simulink library "ET3036TU_model_library_2020a_fix"  (R2020a)
settings: Solver=VariableStepAuto  StartTime=0.0  StopTime=10.0  RelTol=1e-3
values from neighbouring files (symbols this model uses):
  Data =     [Data.mat]
libraries: powerlib x21, simulink x13, powerlib_meascontrol x4
settings Model: Creator=Hazem  LastModifiedBy=simon
settings DebuggingCC: ArithmeticOperatorsInVariantConditions=warning
settings SFSimCC: CustomCodeUndefinedFunction=UseInterfaceOnly

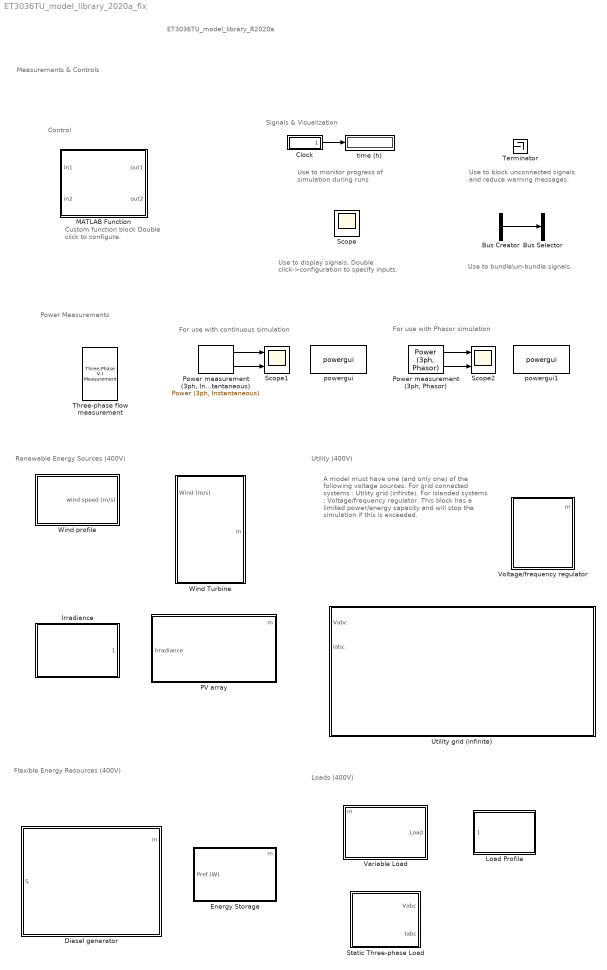
== system ET3036TU_model_library_2020a_fix ==
  note: Flexible Energy Resources (400V)
  note: Signals & Visualization
  note: Control
  note: Power Measurements
  note: ET3036TU_model_library_R2020a
  note: A model must have one (and only one) of the following voltage sources:
      |
      | For grid connected systems : Utility grid (infinite).
      |
      | For islanded systems : Voltage/frequency regulator. This block has a limited power/energy capacity and will stop the simulation if this is exceeded.
  note: Loads (400V)
  note: Utility (400V)
  note: Custom function block
      | Double click to configure.
  note: Use to display signals.
      | Double click->configuration to specify inputs.
  note: Use to bundle\un-bundle signals.
  note: Use to block unconnected signals
      | and reduce warning messages.
  note: Measurements & Controls
  note: Renewable Energy Sources (400V)
  note: For use with Phasor simulation
  note: For use with continuous simulation
  note: Use to monitor progress of
      | simulation during runs
  Bus Creator : BusCreator  Inputs=2
  Bus Selector : BusSelector  OutputSignals=Active power P (W),Reactive power Q (var)
  Clock : Subsystem
  Diesel generator : Subsystem  mask(Controllable Power Plant){Snom=15, Vnom=230*sqrt(3), fnom=50, Pfactor=1}
      mask prompts: Snom "Rated Power (MVA)"; Vnom "Rated phase-to-phase voltage (Vrms)"; fnom "Frequency (Hz)"; Pfactor "Power Factor (leading)"
      mask help: Implements a controllable (dispatchable) power plant with the required governer and excitation subsystems.
      mask Display:
      | image(imread('diesel.jpg'))
      | 
      | color('white')
      | port_label('RConn',1,'A')
      | port_label('RConn',2,'B')
      | port_label('RConn',3,'C')
      | port_label('output',1,'m')
      | 
      | color('black')
      | port_label('input',1,'  Sref (VA)')
  Energy Storage : Subsystem  mask(Grid-connected Energy Storage (PQ Model)){Vn=230*sqrt(3), Fn=50, PnomkW=100, kWh_Rated=500, Efficiency=96, LimitVec=[100 0], RechargeSOC=50, Precharge=100, autoRecharge=off, Initial_kWh_pc=50, PQvec=[0 0]}
      mask prompts: Vn "Nominal L-L Voltage [Vrms]"; Fn "Nominal Frequency [Hz]"; PnomkW "Rated Power [kW]"; kWh_Rated "Rated Capacity [kWh]"; Efficiency "Overall System Efficiency [%]"; LimitVec "Upper/Lower Charge Limits [%]"; RechargeSOC "SOC to Recharge [%]"; Precharge "Recharge Rate [% of Rated Power]"; autoRecharge "Enable Auto-Recharge"; Initial_kWh_pc "Initial State-of-Charge [0-100%]"; PQvec "Initial Active/Reactive Cmds"
      mask help:
      | The energy storage block models a generic grid-connected energy storage system (ESS), most commonly a battery system. This is a system-level model that does not contain any power electronics, but is useful for load flow, phasor, and hybrid phasor-EMT simulations. The inputs to this block are the commanded active and reactive power of the ESS.
      |
      | Note: Positive cmd indicates discharging (supply), negative cmd indicates charging (load).
      | Note: The initial active/reactive power commands must be specified for use for Load Flow analysis.
      mask init:
      | % Calculate Initial Conditions
      | Pnom = PnomkW*1e3;
      | P0 = -PQvec(1);  Q0 = -PQvec(2);
      | if abs(P0) > Pnom
      |     P0 = sign(P0)*Pnom;
      | end
      | 
      | % Calculate Q0 given Reactive Power Capability Curve
      | Qlim = sqrt(Pnom^2 - P0^2);
      | if Qlim > abs(Q0)
      |     Q0 = sign(Q0)*Qlim;
      | end
      | 
      | UpChrgLim = LimitVec(1);
      | LowChrgLim = LimitVec(2);
      | if Initial_kWh_pc > UpChrgLim && P0 < 0
      |     P0 = 0; Q0 = 0;
      | elseif Initial_kWh_pc < LowChrgLim && P0 > 0
      |     P0 = 0; Q0 = 0;
      | end
      mask DialogControl Container7 Prompt: Grid Connection Properties
      mask DialogControl Container11 Prompt: Charge/Discharge Controls
      mask DialogControl Container12 Prompt: Initial Conditions
      mask Display: image(imread('Battery.jpg'))
  Irradiance : Subsystem  mask(Irradiance profile){}
      mask help:
      | Automatically loads irradiance values from the local file 'Data.mat' (variable Data.solar).
      |
      | Expects hourly input irradiance values (W/m2).
      mask init:
      | load Data
      mask Display: plot(Data.solar.hour,Data.solar.direct+Data.solar.diffuse)
  Load Profile : Subsystem
      mask init:
      | load Data
      mask DialogControl DescGroupVar Prompt: Load Profile
      mask DialogControl DescTextVar Prompt: Automatically loads Consumption values from the local file 'Data.mat' (variable Data.varload).
      mask DialogControl Control2 Prompt: Expects per-minute active power consumption values (W).
      mask Display: plot(Data.varload.minute,Data.varload.load)
  MATLAB Function : MATLAB Function  TreatAsAtomicUnit=on
  "PV array " : Subsystem  mask(PV farm){Efficiency=0.2, Area=100, Vnom=230*sqrt(3), fnom=50}
      mask prompts: Efficiency "Total efficiency (fraction)"; Area "Area (m2)"; Vnom "Rated phase-to-phase voltage (Vrms)"; fnom "Rated frequency (Hz):"
      mask help: The product of the efficiency, the area covered by the PV farm and the irradiance in W/m2 will give you the power generated by the PV farm.
      mask Display:
      | color('white')
      | image(imread('pv.jpg'))
      | 
      | color('black')
      | port_label('RConn',1,'A')
      | port_label('RConn',2,'B')
      | port_label('RConn',3,'C')
      | port_label('output',1,'m')
      | 
      | port_label('input',1,'Irradiance (W/m2)')
  "Power measurement (3ph, Instantaneous)" : powerlib_meascontrol/Measurements/Power (3ph, Instantaneous)
  "Power measurement (3ph, Phasor)" : powerlib_meascontrol/Measurements/Power (3ph, Phasor)
      settings: SourceProductBaseCode=PS
  Scope : Scope  NumInputPorts=2
  Scope1 : Scope  NumInputPorts=2
  Scope2 : Scope  NumInputPorts=2
  Static Three-phase Load : Subsystem  mask(Static Three-phase Load){Vnom=230*sqrt(3), fnom=50, Prated=100}
      mask prompts: Vnom "Nominal phase-to-phase voltage Vn (Vrms)"; fnom "Nominal frequency fn (Hz):"; Prated "Active power P (kW):"
      mask help:
      | Implements a three-phase resistive load.
      |
      | Adjust nominal voltage and frequency according to system configuration.
      |
      | Specify rated power consumption.
      mask Display: image(imread('Res.jpg'))
  Terminator : Terminator
  Three-phase flow measurement : powerlib/Measurements/Three-Phase V-I Measurement  VoltageMeasurement=phase-to-ground  SetLabelV=off  LabelV=Vabc  Vpu=off  VpuLL=off  CurrentMeasurement=yes  SetLabelI=off  LabelI=Iabc  Ipu=off  Pbase=100e6  Vbase=500e3  OutputType=Complex  PhasorSimulation=on  PSBequivalent=0
  Utility grid (infinite) : Subsystem  mask(Utility Distribution Substation){Vgrid=230*sqrt(3), fnom=50}
      mask prompts: Vgrid "Grid phase-to-phase  voltage (Vrms)"; fnom "Nominal frequency (Hz):"
      mask help:
      | Implements a grid connection with finite capacity.
      |
      | Supports two-way power flow, set voltages and frequency according to system configuration.
      |
      | Adjust Nominal Power.
      mask Display:
      | image(imread('powersystem.jpg'))
      | 
      | color('white')
      | port_label('RConn',1,'A')
      | port_label('RConn',2,'B')
      | port_label('RConn',3,'C')
      | port_label('output',1,'Vabc')
      | port_label('output',2,'Iabc')
  Variable Load : Subsystem  mask(Variable Load (PQ Model)){Vn=230*sqrt(3), Fn=50, PF=1, Load0=0}
      mask prompts: Vn "Nominal L-L Voltage [Vrms]"; Fn "Nominal Frequency [Hz]"; PF "Power Factor [0 to 1]"; Load0 "Initial Load [W]"
      mask help:
      | The Variable Load block is a lumped approximation for a distribution feeder. For non-unity power factor loads, the input (active power) is scaled accordingly to generate a desired load.
      |
      | Note: The initial input load must be specified for use for Load Flow analysis.
      mask init:
      | P0 = Load0;
      | Q0 = Load0*sqrt(1/PF-1);
      mask Display:
      | image(imread('Residential.jpg'))
      | color('white')
      | port_label('input',1,'Load (W)')
      | port_label('output',1,'m')
      | port_label('Rconn',1,'A')
      | port_label('Rconn',2,'B')
      | port_label('Rconn',3,'C')
  Voltage/frequency regulator : Subsystem  mask{E_max=1e3, Vnom=230*sqrt(3), fnom=50}
      mask prompts: E_max "Rated energy reserve (Wh)"; Vnom "Nominal L-L Voltage (Vrms)"; fnom "Nominal Frequency (Hz)"
      mask Display: image(imread('powerlib_icon.jpg'))
  "Wind Turbine " : Subsystem  mask{Unom=15, Umax=25, Umin=5, Pselect=1: Simple Cubic Power, fnom=50, Vnom=230*sqrt(3), Pnom=20, rp=5, Cp=16/27, rho=1.225, Uvec=[1:1:30], Pvec=[0,0,0,0,21359.3750000000,58193.5000000000,104316.125000000,157104.500000000,213935.875000000,272187.500000000,329236.625000000,382460.500000000,429236.375000000,466941.500000000,492953.125000000,500000,500000,500000,500000,500000,500000,500000,500000,500000,500000,0,0,0,0,0], Tp=0.1, Tq=1, ReactP=0}
      mask prompts: Unom "Nominal Wind Speed [m/s]"; Umax "Maximum Operating Wind [m/s]"; Umin "Minimum Operating Wind [m/s]"; Pselect "Wind Turbine Power Model"; fnom "Nominal frequency (Hz):"; Vnom "Nominal phae-to-phase voltage (Vrms)"; Pnom "Nominal Power, [kW]"; rp "Blade Radius, r [m]"; Cp "Performance Coefficient, Cp"; rho "Air Density, rho [kg/m^3]"; Uvec "Wind Vec [m/s]"; Pvec "Power Vec [W]"; Tp "Active Power Dynamics, Tp [s]"; Tq "Reactive Power Dynamics, Tq [s]"; ReactP "Reactive Power Percentage [%]"
      mask help:
      | Simple Wind Turbine that serves as an Active and Reactive Power Source depending on the Wind Power Curve.
      |
      | The Wind Turbine Power Curve can be defined by one of three models:
      | 1: Simple cubic power curve
      | 2: Physical wind turbine parameters
      | 3: Look-up table (from a wind turbine data sheet).
      |
      | The 'General' and 'Dynamics' tabs apply to all models.
      mask init:
      | A = pi*rp^2;
      | 
      | if Pselect == 1,
      |     Pmax = Pnom*1e3;
      | elseif Pselect == 2,
      |     Pmax = 1/2*rho*Cp*A*Umax^3;
      | else
      |     Pmax = max(Pvec);
      | end
      | Qmax = (ReactP/100)*Pmax;
      mask TypeOptions Pselect: 1: Simple Cubic Power | 2: Physical parameters | 3: Look-up Fit
      mask DialogControl Container4 Prompt: General
      mask DialogControl Container16 Prompt: Turbine
      mask DialogControl Container10 Prompt: Electrical
      mask DialogControl Container12 Prompt: 1: Cubic
      mask DialogControl Container9 Prompt: 2: Physical
      mask DialogControl Container7 Prompt: 3: Lookup
      mask DialogControl Container8 Prompt: Dynamics
      mask Display:
      | image(imread('eolienne.bmp'))
      | 
      | color('white')
      | port_label('LConn',1,'A')
      | port_label('LConn',2,'B')
      | port_label('LConn',3,'C')
      | 
      | color('blue')
      | port_label('output',1,'m')
      | port_label('input',1,'Wind (m/s)')
  Wind profile : Subsystem  mask(Wind profile){}
      mask help:
      | Automatically loads wind speeds from the local file 'Data.mat' (variable Data.wind).
      |
      | Expects hourly input wind speeds (m/s).
      mask init:
      | load Data
      mask Display: plot(Data.wind.hour,Data.wind.speed)
  powergui : powerlib/powergui  Priority=1  SimulationMode=Discrete  SampleTime=1e-3  frequency=60  Iterations=50  frequencyindice=60  Pbase=100e6  ErrMax=1e-4  UnitsV=kV  UnitsW=MW  buscounter=0  FunctionMessages=off  echomessages=off  EnableUseOfTLC=off  CurrentSourceSwitches=off  DisableSnubberDevices=off  DisableRonSwitches=off  DisableVfSwitches=off  DisplayEquations=off  AutomaticDiscreteSolvers=off  SolverType=Tustin/Backward Euler (TBE)  Interpol=off  ExternalGateDelay=off  methode=off  Ts=100  x0status=blocks  SPID=on  SwTol=0  HookPort=off  NonlinearTolerance=0  nMaxIteration=15  ContinueOnMaxIteration=off  RestoreLinks=warning  ResistiveCurrentMeasurement=off  Frange=[0:2:500]  Ylog=off  Xlog=on  ShowGrid=off  save=off  variable=ZData  structure=0  ZoomFFT=off  StartTime=0.0  cycles=1  DisplayStyle=1  fundamental=60  FreqAxis=off  MaxFrequency=1000  frequencyindicesteady=1  RmsSteady=1  display=off
  powergui1 : powerlib/powergui  Priority=1  SimulationMode=Phasor  SampleTime=50e-6  frequency=50  Iterations=50  frequencyindice=60  Pbase=100e6  ErrMax=1e-4  UnitsV=kV  UnitsW=MW  buscounter=0  FunctionMessages=off  echomessages=off  EnableUseOfTLC=off  CurrentSourceSwitches=off  DisableSnubberDevices=off  DisableRonSwitches=off  DisableVfSwitches=off  DisplayEquations=off  AutomaticDiscreteSolvers=off  SolverType=Tustin/Backward Euler (TBE)  Interpol=off  ExternalGateDelay=off  methode=off  Ts=100  x0status=blocks  SPID=on  SwTol=0  HookPort=off  NonlinearTolerance=0  nMaxIteration=15  ContinueOnMaxIteration=off  RestoreLinks=warning  ResistiveCurrentMeasurement=off  Frange=[0:2:500]  Ylog=off  Xlog=on  ShowGrid=off  save=off  variable=ZData  structure=0  ZoomFFT=off  StartTime=0.0  cycles=1  DisplayStyle=1  fundamental=60  FreqAxis=off  MaxFrequency=1000  frequencyindicesteady=1  RmsSteady=1  display=off
  time (h) : Display
      settings: Format=bank
  wires:
  "Power measurement (3ph, Phasor)"/1 -> Scope2/1
  "Power measurement (3ph, Phasor)"/2 -> Scope2/2
  "Power measurement (3ph, Instantaneous)"/1 -> Scope1/1
  "Power measurement (3ph, Instantaneous)"/2 -> Scope1/2
  Clock/1(" ") -> time (h)/1
  Bus Creator/1 -> Bus Selector/1

== system ET3036TU_model_library_2020a_fix/Clock ==
  Clock : Clock
  Gain : Gain  Gain=1/(60*60)
  " " : Outport  VectorParamsAs1DForOutWhenUnconnected=off
  wires:
  Gain/1 -> " "/1
  Clock/1 -> Gain/1

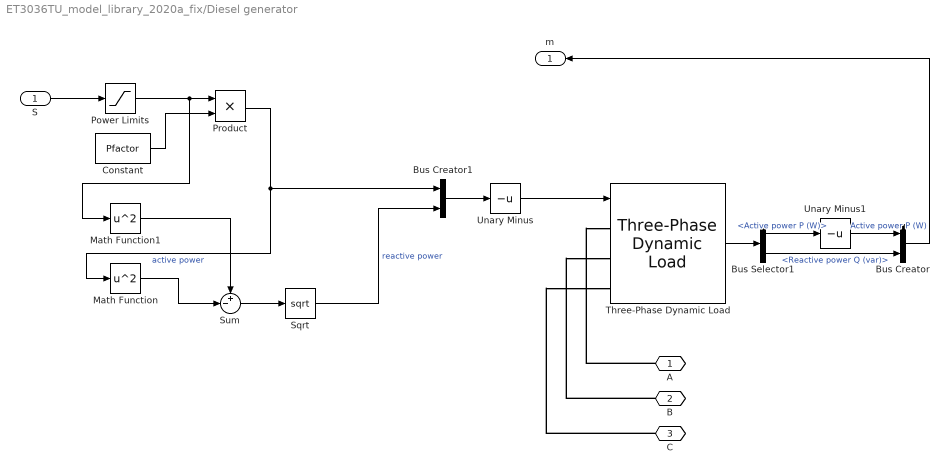
== system ET3036TU_model_library_2020a_fix/Diesel generator ==
  S : Inport
  Bus Creator : BusCreator  Inputs=2
  Bus Creator1 : BusCreator  Inputs=2
  Bus Selector1 : BusSelector  OutputSignals=Active power P (W),Reactive power Q (var)
  Constant : Constant  Value=Pfactor
  Math Function : Math  Operator=square  SignedPower=on  SaturateOnIntegerOverflow=on
  Math Function1 : Math  Operator=square  SignedPower=on  SaturateOnIntegerOverflow=on
  Power Limits : Saturate  UpperLimit=Snom*1e6  LowerLimit=0
  Product : Product
  Sqrt : Sqrt  SaturateOnIntegerOverflow=on
  Sum : Sum  Inputs=+-|
  Three-Phase Dynamic Load : powerlib/Elements/Three-Phase Dynamic Load  NominalVoltage=[Vnom fnom]  ActiveReactivePowers=[0 0]  PositiveSequence=[Vnom 0]  ExternalControl=on  NpNq=[1.3 2]  TimeConstants="[0  0  0  0]"  MinimumVoltage=0.7  Tfilter=1e-4  LoadFlowParameters=[4,0,0,0,0]
      settings: SourceProductBaseCode=PS
  Unary Minus : UnaryMinus
  Unary Minus1 : UnaryMinus
  A : PMIOPort  Side=Right
  B : PMIOPort  Port=2  Side=Right
  C : PMIOPort  Port=3  Side=Right
  m : Outport  VectorParamsAs1DForOutWhenUnconnected=off
  wires:
  Constant/1 -> Product/2
  Math Function1/1 -> Sum/1
  Math Function/1 -> Sum/2
  Product/1 -> Math Function/1, Bus Creator1/1  "active power"
  S/1 -> Power Limits/1
  Sum/1 -> Sqrt/1
  Power Limits/1 -> Math Function1/1, Product/1
  Sqrt/1 -> Bus Creator1/2  "reactive power"
  Bus Selector1/2 -> Bus Creator/2  "<Reactive power Q (var)>"
  Three-Phase Dynamic Load/1 -> Bus Selector1/1
  Bus Selector1/1 -> Unary Minus1/1  "<Active power P (W)>"
  Unary Minus1/1 -> Bus Creator/1  "Active power P (W)"
  Bus Creator/1 -> m/1
  Bus Creator1/1 -> Unary Minus/1
  Unary Minus/1 -> Three-Phase Dynamic Load/1
  connections:
  A/RConn1 -- Three-Phase Dynamic Load/LConn1
  B/RConn1 -- Three-Phase Dynamic Load/LConn2
  C/RConn1 -- Three-Phase Dynamic Load/LConn3

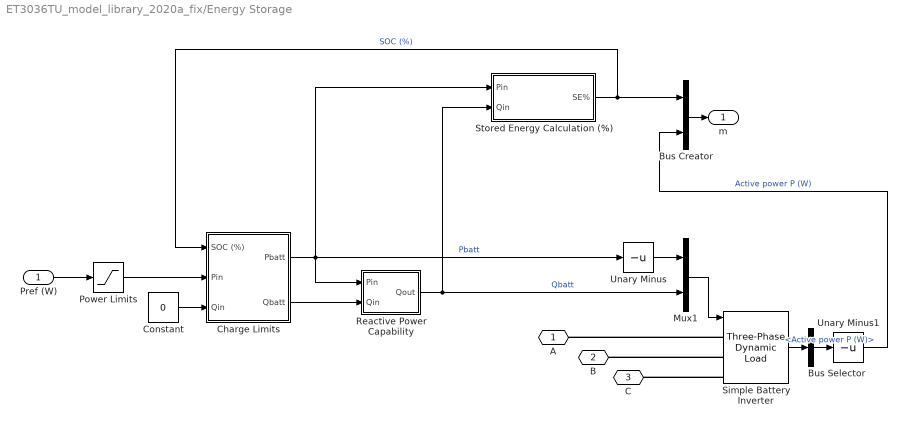
== system ET3036TU_model_library_2020a_fix/Energy Storage ==
  Pref (W) : Inport
  Bus Creator : BusCreator  Inputs=2
  Bus Selector : BusSelector  OutputSignals=Active power P (W)
  Charge Limits : Subsystem
  Constant : Constant  Value=0
  Mux1 : Mux  Inputs=2
  Power Limits : Saturate  UpperLimit=Pnom  LowerLimit=-Pnom
  Reactive Power Capability : Subsystem
  Simple Battery Inverter : powerlib/Elements/Three-Phase Dynamic Load  NominalVoltage=[Vn Fn]  ActiveReactivePowers=[0 0]  PositiveSequence=[Vn 0]  ExternalControl=on  NpNq=[1.3 2]  TimeConstants="[0  0  0  0]"  MinimumVoltage=0.7  Tfilter=1e-4  LoadFlowParameters=[4,0,0,0,0]
      settings: SourceProductBaseCode=PS
  Stored Energy Calculation (%) : Subsystem
  Unary Minus : UnaryMinus
  Unary Minus1 : UnaryMinus
  A : PMIOPort  Side=Right
  B : PMIOPort  Port=2  Side=Right
  C : PMIOPort  Port=3  Side=Right
  m : Outport  VectorParamsAs1DForOutWhenUnconnected=off
  wires:
  Unary Minus/1 -> Mux1/1
  Mux1/1 -> Simple Battery Inverter/1
  Simple Battery Inverter/1 -> Bus Selector/1
  Reactive Power Capability/1(Qout) -> Stored Energy Calculation (%)/2(Qin), Mux1/2  "Qbatt"
  Pref (W)/1 -> Power Limits/1
  Bus Creator/1 -> m/1
  Stored Energy Calculation (%)/1(SE%) -> Charge Limits/1(SOC (%)), Bus Creator/1  "SOC (%)"
  Charge Limits/1(Pbatt) -> Stored Energy Calculation (%)/1(Pin), Unary Minus/1, Reactive Power Capability/1(Pin)  "Pbatt"
  Power Limits/1 -> Charge Limits/2(Pin)
  Constant/1 -> Charge Limits/3(Qin)
  Charge Limits/2(Qbatt) -> Reactive Power Capability/2(Qin)
  Bus Selector/1 -> Unary Minus1/1  "<Active power P (W)>"
  Unary Minus1/1 -> Bus Creator/2  "Active power P (W)"
  connections:
  Simple Battery Inverter/LConn2 -- B/RConn1
  Simple Battery Inverter/LConn3 -- C/RConn1
  Simple Battery Inverter/LConn1 -- A/RConn1

== system ET3036TU_model_library_2020a_fix/Irradiance ==
  Add : Sum
  Add1 : Sum
  Clock1 : Clock
  Constant1 : Constant
  Diffuse irradiance series : Lookup_n-D  NumberOfTableDimensions=1  BreakpointsForDimension1=Data.solar.hour  BeginIndexSearchUsingPreviousIndexResult=on  Table=Data.solar.diffuse  InternalRulePriority=Speed  RndMeth=Simplest  InputSameDT=on
  Direct irradiance series : Lookup_n-D  NumberOfTableDimensions=1  BreakpointsForDimension1=Data.solar.hour  BeginIndexSearchUsingPreviousIndexResult=on  Table=Data.solar.direct  InternalRulePriority=Speed  RndMeth=Simplest  InputSameDT=on
  Second-->Hour : Gain  Gain=1/(60*60)
  " " : Outport  VectorParamsAs1DForOutWhenUnconnected=off
  wires:
  Constant1/1 -> Add/2
  Add/1 -> Direct irradiance series/1, Diffuse irradiance series/1  "Simulation hour"
  Clock1/1 -> Second-->Hour/1
  Second-->Hour/1 -> Add/1
  Diffuse irradiance series/1 -> Add1/1
  Direct irradiance series/1 -> Add1/2
  Add1/1 -> " "/1  "Simulation hour"

== system ET3036TU_model_library_2020a_fix/Load Profile ==
  Add : Sum
  Clock1 : Clock
  Constant1 : Constant
  Second-->Minute : Gain  Gain=1/(60)
  load profile series : Lookup_n-D  NumberOfTableDimensions=1  BreakpointsForDimension1=Data.varload.minute  BeginIndexSearchUsingPreviousIndexResult=on  Table=Data.varload.load  InternalRulePriority=Speed  RndMeth=Simplest  InputSameDT=on
  " " : Outport  VectorParamsAs1DForOutWhenUnconnected=off
  wires:
  Constant1/1 -> Add/2
  Add/1 -> load profile series/1  "Minute"
  load profile series/1 -> " "/1
  Clock1/1 -> Second-->Minute/1
  Second-->Minute/1 -> Add/1

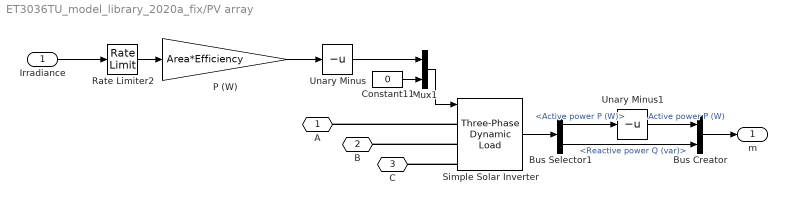
== system ET3036TU_model_library_2020a_fix/PV array  ==
  Irradiance : Inport
  Bus Creator : BusCreator  Inputs=2
  Bus Selector1 : BusSelector  OutputSignals=Active power P (W),Reactive power Q (var)
  Constant11 : Constant  Value=0
  Mux1 : Mux  Inputs=2
  P (W) : Gain  Gain=Area*Efficiency
  Rate Limiter2 : RateLimiter  RisingSlewLimit=1e4  FallingSlewLimit=-1e4  SampleTimeMode=inherited
  Simple Solar Inverter : powerlib/Elements/Three-Phase Dynamic Load  NominalVoltage=[Vnom fnom]  ActiveReactivePowers=[0 0]  PositiveSequence=[Vnom 0]  ExternalControl=on  NpNq=[1.3 2]  TimeConstants="[0  0  0  0]"  MinimumVoltage=0.7  Tfilter=1e-4  LoadFlowParameters=[4,0,0,0,0]
      settings: SourceProductBaseCode=PS
  Unary Minus : UnaryMinus
  Unary Minus1 : UnaryMinus
  A : PMIOPort  Side=Right
  B : PMIOPort  Port=2  Side=Right
  C : PMIOPort  Port=3  Side=Right
  m : Outport  VectorParamsAs1DForOutWhenUnconnected=off
  wires:
  Rate Limiter2/1 -> P (W)/1
  Constant11/1 -> Mux1/2
  Mux1/1 -> Simple Solar Inverter/1
  Unary Minus/1 -> Mux1/1
  Simple Solar Inverter/1 -> Bus Selector1/1
  Bus Selector1/1 -> Unary Minus1/1  "<Active power P (W)>"
  P (W)/1 -> Unary Minus/1
  Irradiance/1 -> Rate Limiter2/1
  Unary Minus1/1 -> Bus Creator/1  "Active power P (W)"
  Bus Selector1/2 -> Bus Creator/2  "<Reactive power Q (var)>"
  Bus Creator/1 -> m/1
  connections:
  Simple Solar Inverter/LConn2 -- B/RConn1
  Simple Solar Inverter/LConn1 -- A/RConn1
  Simple Solar Inverter/LConn3 -- C/RConn1

== system ET3036TU_model_library_2020a_fix/Static Three-phase Load ==
  Static Load : powerlib/Elements/Three-Phase Series RLC Load  LConnTagsString=A|B|C  Configuration=Y (grounded)  NominalVoltage=Vnom  Vabc=[1e3 1e3 1e3]  Vabcp=[1e3 1e3 1e3]  NominalFrequency=fnom  UnbalancedPower=off  ActivePower=Prated*1e3  InductivePower=0  CapacitivePower=0  Pabc=[10e3 9e3 11e3]  QLabc=[100 90 110]  QCabc=[100 90 110]  Pabcp=[10e3 9e3 11e3]  QLabcp=[100 90 110]  QCabcp=[100 90 110]  Measurements=None  LoadType=constant Z
  V-I Measurement : powerlib/Measurements/Three-Phase V-I Measurement  VoltageMeasurement=phase-to-ground  SetLabelV=off  LabelV=Vabc  Vpu=off  VpuLL=off  CurrentMeasurement=yes  SetLabelI=off  LabelI=Iabc  Ipu=off  Pbase=100e6  Vbase=500e3  OutputType=Complex  PhasorSimulation=on  PSBequivalent=0
  A : PMIOPort  Side=Left
  B : PMIOPort  Port=2  Side=Left
  C : PMIOPort  Port=3  Side=Left
  Vabc : Outport  VectorParamsAs1DForOutWhenUnconnected=off
  Iabc : Outport  Port=2  VectorParamsAs1DForOutWhenUnconnected=off
  wires:
  V-I Measurement/1 -> Vabc/1
  V-I Measurement/2 -> Iabc/1
  connections:
  Static Load/LConn1 -- V-I Measurement/LConn1
  V-I Measurement/RConn1 -- A/RConn1
  V-I Measurement/LConn2 -- Static Load/LConn2
  V-I Measurement/RConn3 -- C/RConn1
  Static Load/LConn3 -- V-I Measurement/LConn3
  V-I Measurement/RConn2 -- B/RConn1

== system ET3036TU_model_library_2020a_fix/Utility grid (infinite) ==
  AC Voltage Source : powerlib/Electrical Sources/AC Voltage Source  Amplitude=Vgrid*sqrt(2)/sqrt(3)  Phase=0  Frequency=fnom  SampleTime=0  Measurements=None  BusType=swing  Pref=10e3  Qref=0  Qmin=-inf  Qmax=+inf
  AC Voltage Source1 : powerlib/Electrical Sources/AC Voltage Source  Amplitude=Vgrid*sqrt(2)/sqrt(3)  Phase=-120  Frequency=fnom  SampleTime=0  Measurements=None  BusType=swing  Pref=10e3  Qref=0  Qmin=-inf  Qmax=+inf
  AC Voltage Source2 : powerlib/Electrical Sources/AC Voltage Source  Amplitude=Vgrid*sqrt(2)/sqrt(3)  Phase=120  Frequency=fnom  SampleTime=0  Measurements=None  BusType=swing  Pref=10e3  Qref=0  Qmin=-inf  Qmax=+inf
  Ground : powerlib/Elements/Ground  LConnTagsString=a
  V-I Measurement : powerlib/Measurements/Three-Phase V-I Measurement  VoltageMeasurement=phase-to-ground  SetLabelV=off  LabelV=Vabc  Vpu=off  VpuLL=off  CurrentMeasurement=yes  SetLabelI=off  LabelI=Iabc  Ipu=off  Pbase=100e6  Vbase=500e3  OutputType=Complex  PhasorSimulation=off  PSBequivalent=0
  A : PMIOPort  Side=Right
  B : PMIOPort  Port=2  Side=Right
  C : PMIOPort  Port=3  Side=Right
  Vabc : Outport  VectorParamsAs1DForOutWhenUnconnected=off
  Iabc : Outport  Port=2  VectorParamsAs1DForOutWhenUnconnected=off
  wires:
  V-I Measurement/2 -> Iabc/1  "Iabc"
  V-I Measurement/1 -> Vabc/1  "Vabc"
  connections:
  Ground/LConn1 -- AC Voltage Source2/LConn1 -- AC Voltage Source1/LConn1 -- AC Voltage Source/LConn1
  AC Voltage Source1/RConn1 -- V-I Measurement/LConn2
  AC Voltage Source/RConn1 -- V-I Measurement/LConn1
  AC Voltage Source2/RConn1 -- V-I Measurement/LConn3
  B/RConn1 -- V-I Measurement/RConn2
  C/RConn1 -- V-I Measurement/RConn3
  V-I Measurement/RConn1 -- A/RConn1

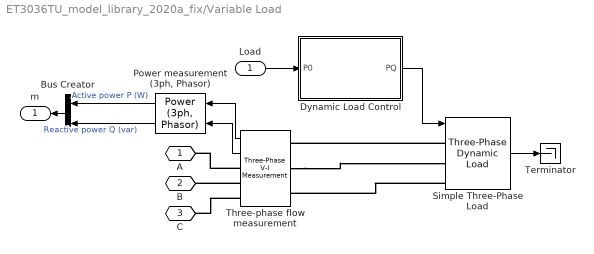
== system ET3036TU_model_library_2020a_fix/Variable Load ==
  Load : Inport
  Bus Creator : BusCreator  Inputs=2
  Dynamic Load Control : Subsystem
  "Power measurement (3ph, Phasor)" : powerlib_meascontrol/Measurements/Power (3ph, Phasor)
      settings: SourceProductBaseCode=PS
  Simple Three-Phase Load : powerlib/Elements/Three-Phase Dynamic Load  NominalVoltage=[Vn Fn]  ActiveReactivePowers=[0 0]  PositiveSequence=[Vn 0]  ExternalControl=on  NpNq=[1.3 2]  TimeConstants="[0  0  0  0]"  MinimumVoltage=0.7  Tfilter=1e-4  LoadFlowParameters=[4,0,0,0,0]
      settings: SourceProductBaseCode=PS
  Terminator : Terminator
  Three-phase flow measurement : powerlib/Measurements/Three-Phase V-I Measurement  VoltageMeasurement=phase-to-ground  SetLabelV=off  LabelV=Vabc  Vpu=off  VpuLL=off  CurrentMeasurement=yes  SetLabelI=off  LabelI=Iabc  Ipu=off  Pbase=100e6  Vbase=500e3  OutputType=Complex  PhasorSimulation=on  PSBequivalent=0
  A : PMIOPort  Side=Right
  B : PMIOPort  Port=2  Side=Right
  C : PMIOPort  Port=3  Side=Right
  m : Outport  VectorParamsAs1DForOutWhenUnconnected=off
  wires:
  "Power measurement (3ph, Phasor)"/2 -> Bus Creator/2  "Reactive power Q (var)"
  "Power measurement (3ph, Phasor)"/1 -> Bus Creator/1  "Active power P (W)"
  Bus Creator/1 -> m/1
  Three-phase flow measurement/1 -> "Power measurement (3ph, Phasor)"/1
  Three-phase flow measurement/2 -> "Power measurement (3ph, Phasor)"/2
  Load/1 -> Dynamic Load Control/1(P0)
  Dynamic Load Control/1(PQ) -> Simple Three-Phase Load/1
  Simple Three-Phase Load/1 -> Terminator/1
  connections:
  Three-phase flow measurement/RConn3 -- C/RConn1
  Three-phase flow measurement/RConn2 -- B/RConn1
  Three-phase flow measurement/RConn1 -- A/RConn1
  Simple Three-Phase Load/LConn3 -- Three-phase flow measurement/LConn3
  Simple Three-Phase Load/LConn1 -- Three-phase flow measurement/LConn1
  Three-phase flow measurement/LConn2 -- Simple Three-Phase Load/LConn2

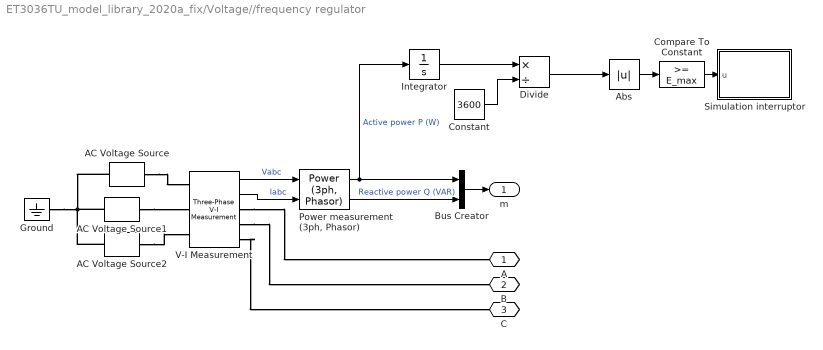
== system ET3036TU_model_library_2020a_fix/Voltage//frequency regulator ==
  AC Voltage Source : powerlib/Electrical Sources/AC Voltage Source  Amplitude=Vnom*sqrt(2)/sqrt(3)  Phase=0  Frequency=fnom  SampleTime=0  Measurements=None  BusType=swing  Pref=10e3  Qref=0  Qmin=-inf  Qmax=+inf
  AC Voltage Source1 : powerlib/Electrical Sources/AC Voltage Source  Amplitude=Vnom*sqrt(2)/sqrt(3)  Phase=-120  Frequency=fnom  SampleTime=0  Measurements=None  BusType=swing  Pref=10e3  Qref=0  Qmin=-inf  Qmax=+inf
  AC Voltage Source2 : powerlib/Electrical Sources/AC Voltage Source  Amplitude=Vnom*sqrt(2)/sqrt(3)  Phase=120  Frequency=fnom  SampleTime=0  Measurements=None  BusType=swing  Pref=10e3  Qref=0  Qmin=-inf  Qmax=+inf
  Abs : Abs
  Bus Creator : BusCreator  Inputs=2
  Compare To Constant : simulink/Logic and Bit Operations/Compare To Constant  relop=>=  const=E_max  OutDataTypeStr=boolean
  Constant : Constant  Value=3600
  Divide : Product  Inputs=*/
  Ground : powerlib/Elements/Ground  LConnTagsString=a
  Integrator : Integrator
  "Power measurement (3ph, Phasor)" : powerlib_meascontrol/Measurements/Power (3ph, Phasor)
      settings: SourceProductBaseCode=PS
  Simulation interruptor : MATLAB Function  TreatAsAtomicUnit=on
  V-I Measurement : powerlib/Measurements/Three-Phase V-I Measurement  VoltageMeasurement=phase-to-ground  SetLabelV=off  LabelV=Vabc  Vpu=off  VpuLL=off  CurrentMeasurement=yes  SetLabelI=off  LabelI=Iabc  Ipu=off  Pbase=100e6  Vbase=500e3  OutputType=Complex  PhasorSimulation=on  PSBequivalent=0
  A : PMIOPort  Side=Right
  B : PMIOPort  Port=2  Side=Right
  C : PMIOPort  Port=3  Side=Right
  m : Outport
  wires:
  "Power measurement (3ph, Phasor)"/1 -> Integrator/1, Bus Creator/1  "Active power P (W)"
  Integrator/1 -> Divide/1
  Abs/1 -> Compare To Constant/1
  V-I Measurement/1 -> "Power measurement (3ph, Phasor)"/1  "Vabc"
  V-I Measurement/2 -> "Power measurement (3ph, Phasor)"/2  "Iabc"
  "Power measurement (3ph, Phasor)"/2 -> Bus Creator/2  "Reactive power Q (VAR)"
  Bus Creator/1 -> m/1
  Compare To Constant/1 -> Simulation interruptor/1(u)
  Constant/1 -> Divide/2
  Divide/1 -> Abs/1
  connections:
  V-I Measurement/RConn3 -- C/RConn1
  AC Voltage Source/RConn1 -- V-I Measurement/LConn1
  AC Voltage Source1/RConn1 -- V-I Measurement/LConn2
  V-I Measurement/RConn1 -- A/RConn1
  AC Voltage Source2/RConn1 -- V-I Measurement/LConn3
  Ground/LConn1 -- AC Voltage Source/LConn1 -- AC Voltage Source1/LConn1 -- AC Voltage Source2/LConn1
  V-I Measurement/RConn2 -- B/RConn1

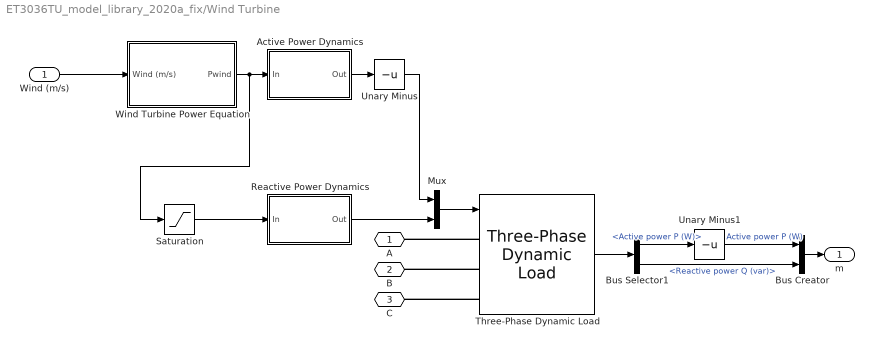
== system ET3036TU_model_library_2020a_fix/Wind Turbine  ==
  Wind (m/s) : Inport
  Active Power Dynamics : Subsystem  VariantControl=T6NotZero
      mask Display: disp('1 / (1 + s T_P)','texmode','on');
  Bus Creator : BusCreator  Inputs=2
  Bus Selector1 : BusSelector  OutputSignals=Active power P (W),Reactive power Q (var)
  Mux : Mux  Inputs=2
  Reactive Power Dynamics : Subsystem  VariantControl=T6NotZero
      mask Display: disp('1 / (1 + s T_Q)','texmode','on');
  Saturation : Saturate  UpperLimit=Qmax  LowerLimit=-Qmax
  Three-Phase Dynamic Load : powerlib/Elements/Three-Phase Dynamic Load  NominalVoltage=[Vnom fnom]  ActiveReactivePowers=[0 0]  PositiveSequence=[Vnom 0]  ExternalControl=on  NpNq=[1.3 2]  TimeConstants="[0  0  0  0]"  MinimumVoltage=0.7  Tfilter=1e-4  LoadFlowParameters=[4,0,0,0,0]
      settings: SourceProductBaseCode=PS
  Unary Minus : UnaryMinus
  Unary Minus1 : UnaryMinus
  Wind Turbine Power Equation : Subsystem
  A : PMIOPort  Side=Left
  B : PMIOPort  Port=2  Side=Left
  C : PMIOPort  Port=3  Side=Left
  m : Outport  VectorParamsAs1DForOutWhenUnconnected=off
  wires:
  Bus Selector1/2 -> Bus Creator/2  "<Reactive power Q (var)>"
  Bus Creator/1 -> m/1
  Unary Minus1/1 -> Bus Creator/1  "Active power P (W)"
  Bus Selector1/1 -> Unary Minus1/1  "<Active power P (W)>"
  Three-Phase Dynamic Load/1 -> Bus Selector1/1
  Unary Minus/1 -> Mux/1
  Active Power Dynamics/1(Out) -> Unary Minus/1
  Wind Turbine Power Equation/1(Pwind) -> Saturation/1, Active Power Dynamics/1(In)
  Mux/1 -> Three-Phase Dynamic Load/1
  Reactive Power Dynamics/1(Out) -> Mux/2
  Saturation/1 -> Reactive Power Dynamics/1(In)
  Wind (m/s)/1 -> Wind Turbine Power Equation/1(Wind (m/s))
  connections:
  Three-Phase Dynamic Load/LConn2 -- B/RConn1
  Three-Phase Dynamic Load/LConn3 -- C/RConn1
  Three-Phase Dynamic Load/LConn1 -- A/RConn1

== system ET3036TU_model_library_2020a_fix/Wind profile ==
  Add : Sum
  Clock1 : Clock
  Constant1 : Constant
  Second-->Hour : Gain  Gain=1/(60*60)
  Wind speed series : Lookup_n-D  NumberOfTableDimensions=1  BreakpointsForDimension1=Data.wind.hour  BeginIndexSearchUsingPreviousIndexResult=on  Table=Data.wind.speed  ExtrapMethod=Clip  UseLastTableValue=on  InternalRulePriority=Speed  RndMeth=Simplest  InputSameDT=on
  wind speed (m/s) : Outport  VectorParamsAs1DForOutWhenUnconnected=off
  wires:
  Second-->Hour/1 -> Add/1
  Add/1 -> Wind speed series/1
  Constant1/1 -> Add/2
  Clock1/1 -> Second-->Hour/1
  Wind speed series/1 -> wind speed (m/s)/1

== system ET3036TU_model_library_2020a_fix/Energy Storage/Charge Limits ==
  SOC (%) : Inport
  Pin : Inport  Port=2
  Qin : Inport  Port=3
  Overcharge Check : Subsystem
  Undercharge Check : Subsystem
  Pbatt : Outport  VectorParamsAs1DForOutWhenUnconnected=off
  Qbatt : Outport  Port=2  VectorParamsAs1DForOutWhenUnconnected=off
  wires:
  Overcharge Check/2(Qout) -> Undercharge Check/3(Qin)
  Undercharge Check/1(Pout) -> Pbatt/1  "Pbatt"
  Qin/1 -> Overcharge Check/3(Qin)
  Overcharge Check/1(Pout) -> Undercharge Check/2(Pin)
  Pin/1 -> Overcharge Check/2(Pin)
  Undercharge Check/2(Qout) -> Qbatt/1
  SOC (%)/1 -> Undercharge Check/1(SOC (%)), Overcharge Check/1(SOC (%))

== system ET3036TU_model_library_2020a_fix/Energy Storage/Reactive Power Capability ==
  Pin : Inport
  Qin : Inport  Port=2
  Constant : Constant  Value=Pnom
  Math Function : Math  Operator=square  SignedPower=on  SaturateOnIntegerOverflow=on
  Math Function1 : Math  Operator=square  SignedPower=on  SaturateOnIntegerOverflow=on
  Saturation Dynamic : simulink/Discontinuities/Saturation Dynamic  OutMin=[]  OutMax=[]  OutDataTypeStr=Inherit: Same as second input  OutDataType=fixdt(1, 16)  OutScaling=2^-10  DoSatur=off
  Sqrt : Sqrt  SaturateOnIntegerOverflow=on
  Sum : Sum  Inputs=-+|
  Unary Minus : UnaryMinus
  Qout : Outport  VectorParamsAs1DForOutWhenUnconnected=off
  wires:
  Qin/1 -> Saturation Dynamic/2
  Pin/1 -> Math Function1/1
  Saturation Dynamic/1 -> Qout/1
  Unary Minus/1 -> Saturation Dynamic/3
  Sum/1 -> Sqrt/1
  Constant/1 -> Math Function/1
  Math Function/1 -> Sum/2
  Math Function1/1 -> Sum/1
  Sqrt/1 -> Unary Minus/1, Saturation Dynamic/1

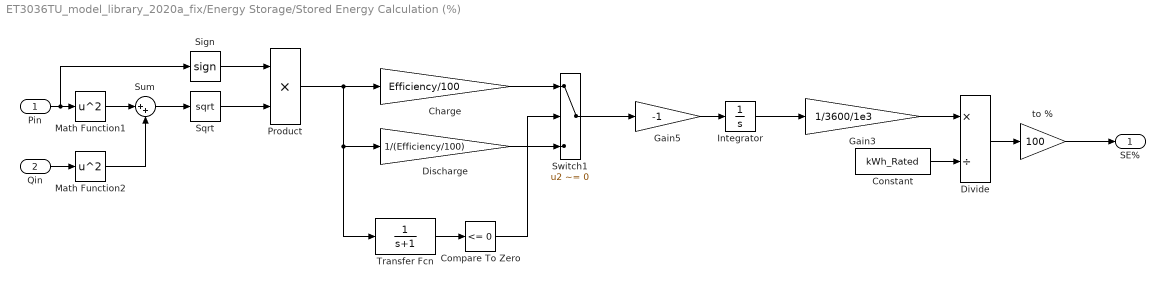
== system ET3036TU_model_library_2020a_fix/Energy Storage/Stored Energy Calculation (%) ==
  Pin : Inport
  Qin : Inport  Port=2
  Charge : Gain  Gain=Efficiency/100
  Compare To Zero : simulink/Logic and Bit Operations/Compare To Zero  relop=<=  OutDataTypeStr=boolean
  Constant : Constant  Value=kWh_Rated
  Discharge : Gain  Gain=1/(Efficiency/100)
  Divide : Product  Inputs=*/
  Gain3 : Gain  Gain=1/3600/1e3
  Gain5 : Gain  Gain=-1
  Integrator : Integrator  InitialCondition=(Initial_kWh_pc/100)*kWh_Rated*3600*1e3
  Math Function1 : Math  Operator=square  SignedPower=on  SaturateOnIntegerOverflow=on
  Math Function2 : Math  Operator=square  SignedPower=on  SaturateOnIntegerOverflow=on
  Product : Product
  Sign : Signum
  Sqrt : Sqrt  SaturateOnIntegerOverflow=on
  Sum : Sum  Inputs=|++
  Switch1 : Switch  Criteria=u2 ~= 0
  Transfer Fcn : TransferFcn  Denominator=[1 1]
  to % : Gain  Gain=100
  SE% : Outport  VectorParamsAs1DForOutWhenUnconnected=off
  wires:
  Integrator/1 -> Gain3/1
  Compare To Zero/1 -> Switch1/2
  Divide/1 -> to %/1
  Charge/1 -> Switch1/1
  Constant/1 -> Divide/2
  Gain3/1 -> Divide/1
  Switch1/1 -> Gain5/1
  Transfer Fcn/1 -> Compare To Zero/1
  to %/1 -> SE%/1
  Gain5/1 -> Integrator/1
  Discharge/1 -> Switch1/3
  Product/1 -> Charge/1, Discharge/1, Transfer Fcn/1
  Pin/1 -> Sign/1, Math Function1/1
  Qin/1 -> Math Function2/1
  Math Function1/1 -> Sum/1
  Math Function2/1 -> Sum/2
  Sum/1 -> Sqrt/1
  Sqrt/1 -> Product/2
  Sign/1 -> Product/1

== system ET3036TU_model_library_2020a_fix/Variable Load/Dynamic Load Control ==
  P0 : Inport
  Fcn : Fcn  Expr=sqrt(1/u(1)-1)
  Mux : Mux  Inputs=2
  Product : Product
  Summer1 : Constant  Value=PF
  PQ : Outport  VectorParamsAs1DForOutWhenUnconnected=off
  wires:
  Summer1/1 -> Fcn/1
  Fcn/1 -> Product/2
  P0/1 -> Product/1, Mux/1
  Mux/1 -> PQ/1
  Product/1 -> Mux/2  "Qo"

== system ET3036TU_model_library_2020a_fix/Wind Turbine /Active Power Dynamics ==
  In : Inport
  1/Tp : Gain  Gain=1/Tp
  Integrator : Integrator
  Sum : Sum  Inputs=|+-
  Out : Outport  VectorParamsAs1DForOutWhenUnconnected=off
  wires:
  Integrator/1 -> Out/1, Sum/2
  In/1 -> Sum/1
  1/Tp/1 -> Integrator/1
  Sum/1 -> 1/Tp/1

== system ET3036TU_model_library_2020a_fix/Wind Turbine /Reactive Power Dynamics ==
  In : Inport
  1/Tq : Gain  Gain=1/Tq
  Integrator : Integrator
  Sum : Sum  Inputs=|+-
  Out : Outport  VectorParamsAs1DForOutWhenUnconnected=off
  wires:
  Sum/1 -> 1/Tq/1
  1/Tq/1 -> Integrator/1
  In/1 -> Sum/1
  Integrator/1 -> Sum/2, Out/1

== system ET3036TU_model_library_2020a_fix/Wind Turbine /Wind Turbine Power Equation ==
  Wind (m/s) : Inport
  Constant : Constant  Value=Pselect
  Cubic Power with Cutoff : Subsystem
  Manufacturer Fit : Lookup_n-D  NumberOfTableDimensions=1  BreakpointsForDimension1=Uvec  Table=Pvec  ExtrapMethod=Clip  InternalRulePriority=Speed  RndMeth=Simplest  InputSameDT=on
  Multiport Switch : MultiPortSwitch
  Saturation : Saturate  UpperLimit=inf  LowerLimit=0  ZeroCross=off
      settings: AttributesFormatString=|
      | %<UpperLimit>
      | %<LowerLimit>
  Wind Turbine Properties : Subsystem
  Pwind : Outport  VectorParamsAs1DForOutWhenUnconnected=off
  wires:
  Manufacturer Fit/1 -> Multiport Switch/4
  Saturation/1 -> Manufacturer Fit/1, Wind Turbine Properties/1(Wind (m/s)), Cubic Power with Cutoff/1(Wind (m/s))
  Constant/1 -> Multiport Switch/1
  Multiport Switch/1 -> Pwind/1
  Wind (m/s)/1 -> Saturation/1
  Wind Turbine Properties/1(Pwind) -> Multiport Switch/3
  Cubic Power with Cutoff/1(Pwind) -> Multiport Switch/2

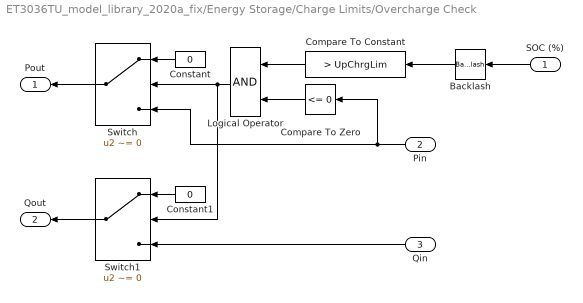
== system ET3036TU_model_library_2020a_fix/Energy Storage/Charge Limits/Overcharge Check ==
  SOC (%) : Inport
  Pin : Inport  Port=2
  Qin : Inport  Port=3
  Backlash : Backlash  BacklashWidth=1e-3  InitialOutput=Initial_kWh_pc  ZeroCross=off
  Compare To Constant : simulink/Logic and Bit Operations/Compare To Constant  relop=>  const=UpChrgLim  OutDataTypeStr=boolean
  Compare To Zero : simulink/Logic and Bit Operations/Compare To Zero  relop=<=  OutDataTypeStr=boolean
  Constant : Constant  Value=0
  Constant1 : Constant  Value=0
  Logical Operator : Logic  AllPortsSameDT=off  OutDataTypeStr=boolean
  Switch : Switch  Criteria=u2 ~= 0
  Switch1 : Switch  Criteria=u2 ~= 0
  Pout : Outport  VectorParamsAs1DForOutWhenUnconnected=off
  Qout : Outport  Port=2  VectorParamsAs1DForOutWhenUnconnected=off
  wires:
  Compare To Constant/1 -> Logical Operator/1
  Logical Operator/1 -> Switch1/2, Switch/2
  Constant/1 -> Switch/1
  SOC (%)/1 -> Backlash/1
  Pin/1 -> Compare To Zero/1, Switch/3
  Switch/1 -> Pout/1
  Compare To Zero/1 -> Logical Operator/2
  Qin/1 -> Switch1/3
  Constant1/1 -> Switch1/1
  Switch1/1 -> Qout/1
  Backlash/1 -> Compare To Constant/1

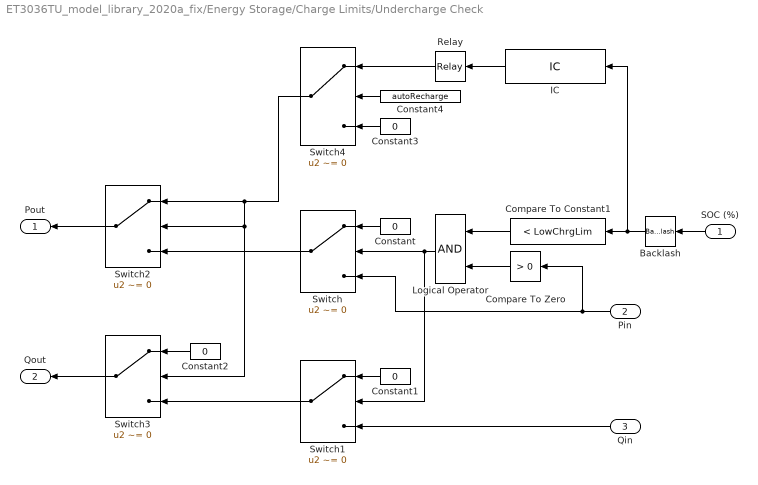
== system ET3036TU_model_library_2020a_fix/Energy Storage/Charge Limits/Undercharge Check ==
  SOC (%) : Inport
  Pin : Inport  Port=2
  Qin : Inport  Port=3
  Backlash : Backlash  BacklashWidth=1e-3  InitialOutput=Initial_kWh_pc  ZeroCross=off
  Compare To Constant1 : simulink/Logic and Bit Operations/Compare To Constant  relop=<  const=LowChrgLim  OutDataTypeStr=boolean
  Compare To Zero : simulink/Logic and Bit Operations/Compare To Zero  relop=>  OutDataTypeStr=boolean
  Constant{,1..3} (4 alike) : Constant  Value=0
  Constant4 : Constant  Value=autoRecharge
  IC : InitialCondition  Value=RechargeSOC
  Logical Operator : Logic  AllPortsSameDT=off  OutDataTypeStr=boolean
  Relay : Relay  OnSwitchValue=RechargeSOC  OffSwitchValue=LowChrgLim  OnOutputValue=0  OffOutputValue=-Precharge/100*Pnom
  Switch{,1..4} (5 alike) : Switch  Criteria=u2 ~= 0
  Pout : Outport  VectorParamsAs1DForOutWhenUnconnected=off
  Qout : Outport  Port=2  VectorParamsAs1DForOutWhenUnconnected=off
  wires:
  Compare To Zero/1 -> Logical Operator/2
  Pin/1 -> Switch/3, Compare To Zero/1
  SOC (%)/1 -> Backlash/1
  Constant/1 -> Switch/1
  Logical Operator/1 -> Switch/2, Switch1/2
  Compare To Constant1/1 -> Logical Operator/1
  Constant1/1 -> Switch1/1
  Qin/1 -> Switch1/3
  Backlash/1 -> IC/1, Compare To Constant1/1
  Switch4/1 -> Switch2/1, Switch2/2, Switch3/2
  IC/1 -> Relay/1
  Switch/1 -> Switch2/3
  Switch2/1 -> Pout/1
  Switch3/1 -> Qout/1
  Switch1/1 -> Switch3/3
  Constant2/1 -> Switch3/1
  Relay/1 -> Switch4/1
  Constant3/1 -> Switch4/3
  Constant4/1 -> Switch4/2

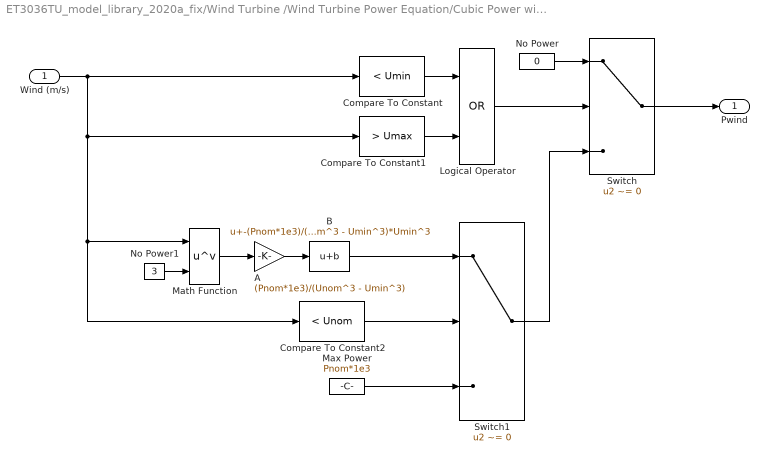
== system ET3036TU_model_library_2020a_fix/Wind Turbine /Wind Turbine Power Equation/Cubic Power with Cutoff ==
  Wind (m/s) : Inport
  A : Gain  Gain=(Pnom*1e3)/(Unom^3 - Umin^3)
  B : Bias  Bias=-(Pnom*1e3)/(Unom^3 - Umin^3)*Umin^3
  Compare To Constant : simulink/Logic and Bit Operations/Compare To Constant  relop=<  const=Umin  OutDataTypeStr=boolean
  Compare To Constant1 : simulink/Logic and Bit Operations/Compare To Constant  relop=>  const=Umax  OutDataTypeStr=boolean
  Compare To Constant2 : simulink/Logic and Bit Operations/Compare To Constant  relop=<  const=Unom  OutDataTypeStr=boolean
  Logical Operator : Logic  Operator=OR  AllPortsSameDT=off  OutDataTypeStr=boolean
  Math Function : Math  Operator=pow  SignedPower=on  SaturateOnIntegerOverflow=on
  Max Power : Constant  Value=Pnom*1e3
  No Power : Constant  Value=0
  No Power1 : Constant  Value=3
  Switch : Switch  Criteria=u2 ~= 0  ZeroCross=off
  Switch1 : Switch  Criteria=u2 ~= 0  ZeroCross=off
  Pwind : Outport  VectorParamsAs1DForOutWhenUnconnected=off
  wires:
  Compare To Constant/1 -> Logical Operator/1
  Switch/1 -> Pwind/1
  Logical Operator/1 -> Switch/2
  A/1 -> B/1
  Wind (m/s)/1 -> Compare To Constant2/1, Math Function/1, Compare To Constant1/1, Compare To Constant/1
  Max Power/1 -> Switch1/3
  Switch1/1 -> Switch/3
  No Power/1 -> Switch/1
  No Power1/1 -> Math Function/2
  Math Function/1 -> A/1
  Compare To Constant1/1 -> Logical Operator/2
  Compare To Constant2/1 -> Switch1/2
  B/1 -> Switch1/1

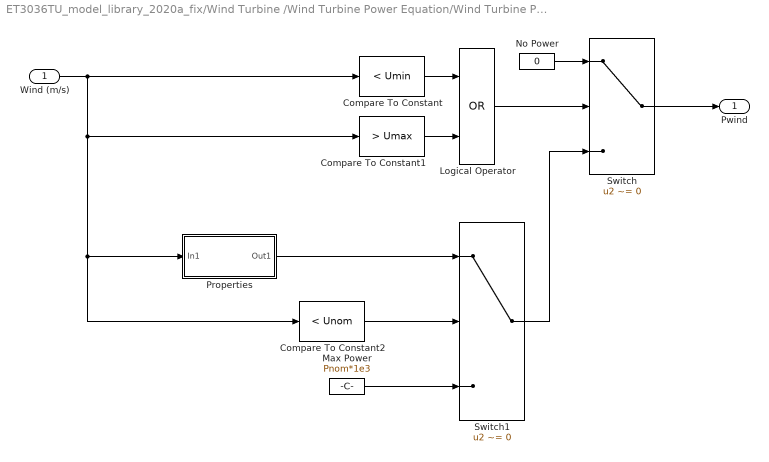
== system ET3036TU_model_library_2020a_fix/Wind Turbine /Wind Turbine Power Equation/Wind Turbine Properties ==
  Wind (m/s) : Inport
  Compare To Constant : simulink/Logic and Bit Operations/Compare To Constant  relop=<  const=Umin  OutDataTypeStr=boolean
  Compare To Constant1 : simulink/Logic and Bit Operations/Compare To Constant  relop=>  const=Umax  OutDataTypeStr=boolean
  Compare To Constant2 : simulink/Logic and Bit Operations/Compare To Constant  relop=<  const=Unom  OutDataTypeStr=boolean
  Logical Operator : Logic  Operator=OR  AllPortsSameDT=off  OutDataTypeStr=boolean
  Max Power : Constant  Value=Pnom*1e3
  No Power : Constant  Value=0
  Properties : Subsystem
  Switch : Switch  Criteria=u2 ~= 0  ZeroCross=off
  Switch1 : Switch  Criteria=u2 ~= 0  ZeroCross=off
  Pwind : Outport  VectorParamsAs1DForOutWhenUnconnected=off
  wires:
  Properties/1(Out1) -> Switch1/1
  Compare To Constant2/1 -> Switch1/2
  Compare To Constant1/1 -> Logical Operator/2
  No Power/1 -> Switch/1
  Switch1/1 -> Switch/3
  Max Power/1 -> Switch1/3
  Wind (m/s)/1 -> Compare To Constant/1, Compare To Constant1/1, Properties/1(In1), Compare To Constant2/1
  Logical Operator/1 -> Switch/2
  Switch/1 -> Pwind/1
  Compare To Constant/1 -> Logical Operator/1

== system ET3036TU_model_library_2020a_fix/Wind Turbine /Wind Turbine Power Equation/Wind Turbine Properties/Properties ==
  In1 : Inport
  Air Density : Gain  Gain=rho
  Blade Swept Area (m^2) : Gain  Gain=A
  Gain : Gain  Gain=1/2
  Power Coefficient : Constant  Value=Cp
  "Product " : Product  SaturateOnIntegerOverflow=on  OutDataTypeStr=Inherit: Same as first input
  wind_speed^3 : Fcn  Expr=u(1)^3
  Out1 : Outport  VectorParamsAs1DForOutWhenUnconnected=off
  wires:
  Blade Swept Area (m^2)/1 -> "Product "/1
  wind_speed^3/1 -> Air Density/1
  Power Coefficient/1 -> "Product "/2
  In1/1 -> wind_speed^3/1
  Air Density/1 -> Gain/1
  "Product "/1 -> Out1/1
  Gain/1 -> Blade Swept Area (m^2)/1

== matlab function ET3036TU_model_library_2020a_fix/MATLAB Function ==
  data: in1 input; out1 output; in2 input; out2 output
function [out1,out2] = Controller(in1,in2)
% An example function that takes two inputs (in1,in2) and gives two output
% (out1,out2)
out1 = in1;
out2 = in2;

== matlab function ET3036TU_model_library_2020a_fix/Voltage//frequency regulator/Simulation interruptor ==
  data: u input
function  fcn(u)
if u==1
    error('Simulation interrupted: System supply/demand imbalance.')
end
